simulink model "Controller_CompareModelWithMeasurement"  (R2019b)
settings: Solver=VariableStepAuto  StartTime=0.0  StopTime=10.0  RelTol=1e-3
values from neighbouring files (symbols this model uses):
  I_init = 0    [PerformExperiment_CompareModelWithMeasurement.m]
  UseUserDefinedBallReference = 1    [LQG_ball.m]    (also in LQG_plate_ball.m; LQR_ball.m; PerformExperiment_CompareModelWithMeasurement.m = 0; Template_PerformExperiment.m = 0)
  UseUserDefinedPlateReference = 1    [LQG_ball.m]    (also in LQG_plate_ball.m; LQR_ball.m; PerformExperiment_CompareModelWithMeasurement.m; Template_PerformExperiment.m = 0)
undefined symbols (not defined in the file or in its folder): denc_mi, numc_mi
settings Model: Creator=Duin home  LastModifiedBy=Duin home

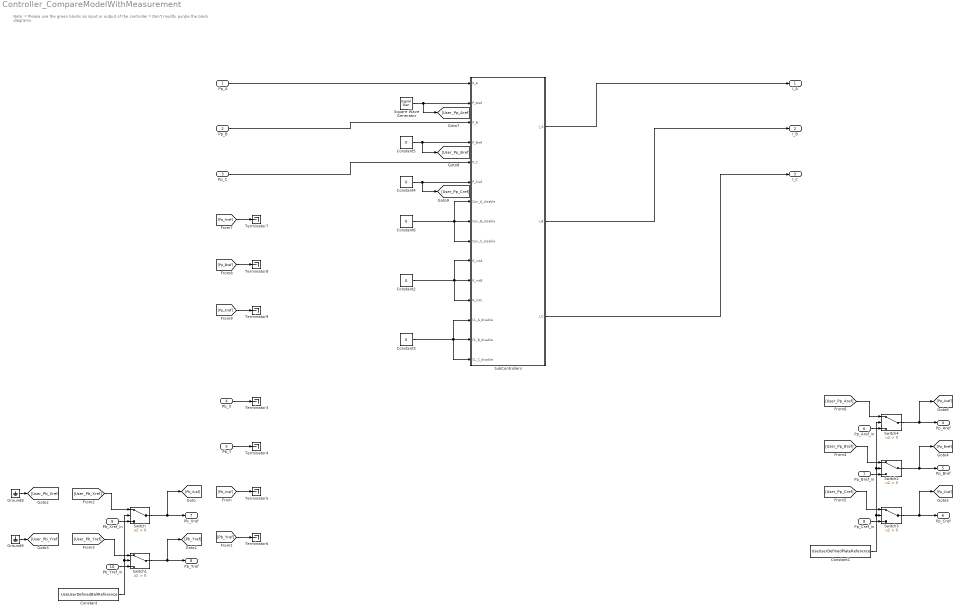
== system Controller_CompareModelWithMeasurement ==
  note: Note:
      | * Please use the green blocks as input or output of the controller
      | * Don't modify purple the block diagrams.
  Pp_A : Inport
  Pp_B : Inport  Port=2
  Pp_C : Inport  Port=3
  Pb_X : Inport  Port=4
  Pb_Y : Inport  Port=5
  Pp_Aref_in : Inport  Port=6
  Pp_Bref_in : Inport  Port=7
  Pp_Cref_in : Inport  Port=8
  Pb_Xref_in : Inport  Port=9
  Pb_Yref_in : Inport  Port=10
  Constant : Constant  Value=UseUserDefinedBallReference
  Constant1 : Constant  Value=UseUserDefinedPlateReference
  Constant{2..6} (5 alike) : Constant  Value=0
  Ground8 : Ground
  Ground9 : Ground
  Square Wave Generator : SignalGenerator  WaveForm=square  Amplitude=0.025  Frequency=0.5  Units=rad/sec
  SubControllers : Subsystem
  Switch{,1..4} (5 alike) : Switch  Criteria=u2 > Threshold
  Terminator{3..9} (7 alike) : Terminator
  I_A : Outport
  I_B : Outport  Port=2
  I_C : Outport  Port=3
  Pp_Aref : Outport  Port=4
  Pp_Bref : Outport  Port=5
  Pp_Cref : Outport  Port=6
  Pb_Xref : Outport  Port=7
  Pb_Yref : Outport  Port=8
  wires:
  Pb_X/1 -> Terminator3/1
  Pb_Y/1 -> Terminator4/1
  SubControllers/2(I_B) -> I_B/1
  SubControllers/1(I_A) -> I_A/1
  Constant4/1 -> [User_Pp_Cref], SubControllers/6(P_Cref)
  Constant5/1 -> [User_Pp_Bref], SubControllers/4("P_Bref ")
  Square Wave Generator/1 -> [User_Pp_Aref], SubControllers/2(P_Aref)
  Pb_Xref_in/1 -> Switch/3
  Pb_Yref_in/1 -> Switch1/3
  Switch1/1 -> [Pb_Yref], Pb_Yref/1
  Switch/1 -> [Pb_Xref], Pb_Xref/1
  [User_Pb_Xref] -> Switch/1
  [User_Pb_Yref] -> Switch1/1
  Constant/1 -> Switch/2, Switch1/2
  Ground8/1 -> [User_Pb_Xref]
  Ground9/1 -> [User_Pb_Yref]
  [Pb_Yref] -> Terminator6/1
  [Pb_Xref] -> Terminator5/1
  Pp_Bref_in/1 -> Switch2/3
  [User_Pp_Bref] -> Switch2/1
  Switch3/1 -> [Pp_Cref], Pp_Cref/1
  Switch2/1 -> [Pp_Bref], Pp_Bref/1
  Pp_Cref_in/1 -> Switch3/3
  Constant1/1 -> Switch4/2, Switch2/2, Switch3/2
  [User_Pp_Cref] -> Switch3/1
  [User_Pp_Aref] -> Switch4/1
  Pp_Aref_in/1 -> Switch4/3
  Switch4/1 -> [Pp_Aref], Pp_Aref/1
  [Pp_Bref] -> Terminator8/1
  [Pp_Aref] -> Terminator7/1
  [Pp_Cref] -> Terminator9/1
  Pp_C/1 -> SubControllers/5(P_C)
  SubControllers/3(I_C) -> I_C/1
  Constant3/1 -> SubControllers/13(CL_A_disable), SubControllers/15(CL_C_disable), SubControllers/14(CL_B_disable)
  Constant2/1 -> SubControllers/11(R_intB), SubControllers/10(R_intA), SubControllers/12(R_intC)
  Constant6/1 -> SubControllers/7(Con_A_disable), SubControllers/9(Con_C_disable), SubControllers/8(Con_B_disable)
  Pp_A/1 -> SubControllers/1(P_A)
  Pp_B/1 -> SubControllers/3(P_B)

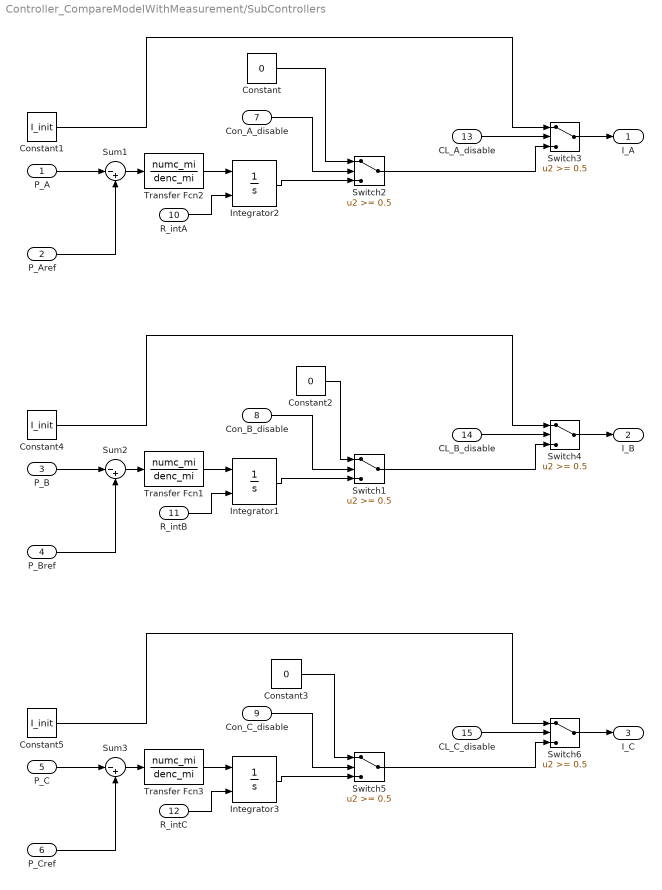
== system Controller_CompareModelWithMeasurement/SubControllers ==
  P_A : Inport
  P_Aref : Inport  Port=2
  P_B : Inport  Port=3
  "P_Bref " : Inport  Port=4
  P_C : Inport  Port=5
  P_Cref : Inport  Port=6
  Con_A_disable : Inport  Port=7
  Con_B_disable : Inport  Port=8
  Con_C_disable : Inport  Port=9
  R_intA : Inport  Port=10
  R_intB : Inport  Port=11
  R_intC : Inport  Port=12
  CL_A_disable : Inport  Port=13
  CL_B_disable : Inport  Port=14
  CL_C_disable : Inport  Port=15
  Constant : Constant  Value=0
  Constant1 : Constant  Value=I_init
  Constant2 : Constant  Value=0
  Constant3 : Constant  Value=0
  Constant4 : Constant  Value=I_init
  Constant5 : Constant  Value=I_init
  Integrator1 : Integrator  ExternalReset=rising  LimitOutput=on  UpperSaturationLimit=3  LowerSaturationLimit=-3
  Integrator2 : Integrator  ExternalReset=rising  LimitOutput=on  UpperSaturationLimit=3  LowerSaturationLimit=-3
  Integrator3 : Integrator  ExternalReset=rising  LimitOutput=on  UpperSaturationLimit=3  LowerSaturationLimit=-3
  Sum1 : Sum  Inputs=|-+  SaturateOnIntegerOverflow=on
  Sum2 : Sum  Inputs=|-+  SaturateOnIntegerOverflow=on
  Sum3 : Sum  Inputs=|-+  SaturateOnIntegerOverflow=on
  Switch{1..6} (6 alike) : Switch  Threshold=0.5
  Transfer Fcn1 : TransferFcn  Numerator=numc_mi  Denominator=denc_mi
  Transfer Fcn2 : TransferFcn  Numerator=numc_mi  Denominator=denc_mi
  Transfer Fcn3 : TransferFcn  Numerator=numc_mi  Denominator=denc_mi
  I_A : Outport
  I_B : Outport  Port=2
  I_C : Outport  Port=3
  wires:
  Switch1/1 -> Switch4/3
  R_intA/1 -> Integrator2/2
  Integrator3/1 -> Switch5/3
  Con_C_disable/1 -> Switch5/2
  Constant5/1 -> Switch6/1
  P_C/1 -> Sum3/1
  Transfer Fcn3/1 -> Integrator3/1
  Switch5/1 -> Switch6/3
  Switch6/1 -> I_C/1
  Sum3/1 -> Transfer Fcn3/1
  Integrator1/1 -> Switch1/3
  Constant1/1 -> Switch3/1
  Constant3/1 -> Switch5/1
  CL_C_disable/1 -> Switch6/2
  R_intC/1 -> Integrator3/2
  Transfer Fcn1/1 -> Integrator1/1
  Sum2/1 -> Transfer Fcn1/1
  Con_B_disable/1 -> Switch1/2
  R_intB/1 -> Integrator1/2
  P_B/1 -> Sum2/1
  Constant2/1 -> Switch1/1
  CL_A_disable/1 -> Switch3/2
  Constant4/1 -> Switch4/1
  CL_B_disable/1 -> Switch4/2
  P_A/1 -> Sum1/1
  P_Aref/1 -> Sum1/2
  Switch2/1 -> Switch3/3
  Constant/1 -> Switch2/1
  Transfer Fcn2/1 -> Integrator2/1
  Switch3/1 -> I_A/1
  Integrator2/1 -> Switch2/3
  Con_A_disable/1 -> Switch2/2
  Sum1/1 -> Transfer Fcn2/1
  P_Cref/1 -> Sum3/2
  "P_Bref "/1 -> Sum2/2
  Switch4/1 -> I_B/1
